simulink model "P1_Ex1"  (R2021a)
settings: Solver=FixedStepAuto  StartTime=0.0  StopTime=Total_time  RelTol=1e-3
PreLoadFcn:
  | PreLoad_P1_Ex1
StopFcn:
  | post_P1_Ex1
values from neighbouring files (symbols this model uses):
  Tg = 0.005    [PreLoad_P1_Ex1.m]
libraries: arduinolib x5, simulink x2
settings Model: SimulationMode=external  ExtModeTrigDuration=2  Creator=Eneko Lerma  LastModifiedBy=Control Automatic
settings SolverCC: AlgebraicLoopSolver=TrustRegion
settings DataIOCC: ReturnWorkspaceOutputs=off
settings OptimizationCC: EnhancedBackFolding=on  PassReuseOutputArgsAs=Individual arguments  MaxStackSize=64  OptimizeBlockOrder=speed  DifferentSizesBufferReuse=on  OptimizationCustomize=off  EfficientTunableParamExpr=on
settings DebuggingCC: ParameterPrecisionLossMsg=none  ParameterTunabilityLossMsg=error  SFMachineParentedDataDiag=warning  ArithmeticOperatorsInVariantConditions=warning
settings HardwareCC: ProdBitPerPointer=32  ProdBitPerSizeT=32  ProdBitPerPtrDiffT=32  ProdLargestAtomicInteger=Long  ProdLargestAtomicFloat=Double  ProdWordSize=32  ProdHWDeviceType=ARM Compatible->ARM Cortex
settings SFSimCC: SimUseLocalCustomCode=off  MATLABDynamicMemAlloc=off  CustomCodeUndefinedFunction=UseInterfaceOnly
settings RTWCC: SystemTargetFile=ert.tlc  HardwareBoard=Arduino Due  TemplateMakefile=ert_default_tmf  GenerateReport=on  RTWUseLocalCustomCode=off  Toolchain=Arduino ARM  BuildConfiguration=Faster Runs  IncludeHyperlinkInReport=on  LaunchReport=on  GenerateTraceInfo=on  GenerateTraceReport=on  GenerateTraceReportSl=on  GenerateTraceReportSf=on  GenerateTraceReportEml=on
settings RTWCC: CustomTerminator=|
  | writeDigitalPin((uint8_T)3, 0);
  | writeDigitalPin((uint8_T)5, 0);
settings CodeAppCC: ForceParamTrailComments=on  IgnoreCustomStorageClasses=off  OperatorAnnotations=on  SimulinkDataObjDesc=on  SFDataObjDesc=on  InsertBlockDesc=on
settings ERTTargetCC: SupportContinuousTime=on  SupportVariableSizeSignals=on

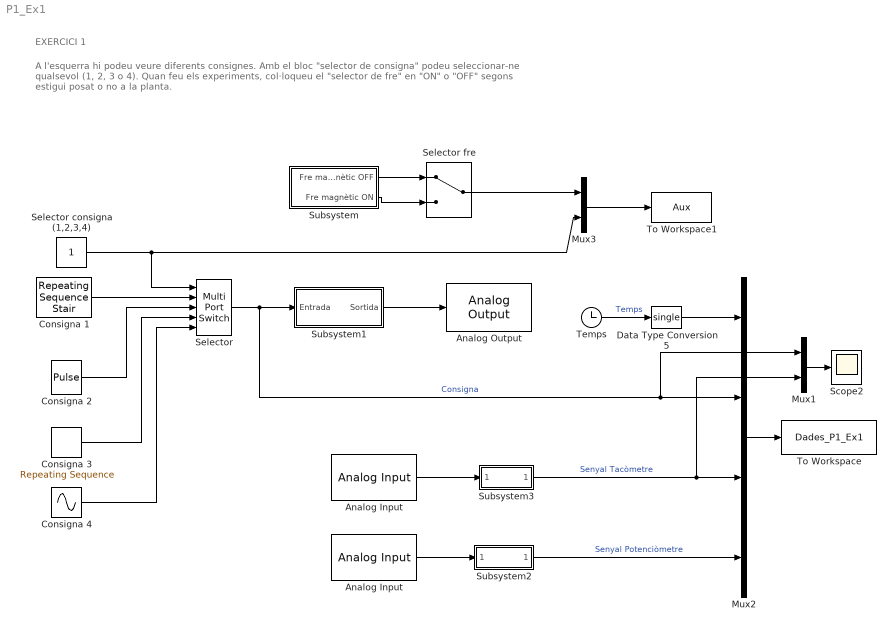
== system P1_Ex1 ==
  note: A l'esquerra hi podeu veure diferents consignes. Amb el bloc "selector de consigna" podeu seleccionar-ne
      | qualsevol (1, 2, 3 o 4). Quan feu els experiments, col·loqueu el "selector de fre" en "ON" o "OFF"
      | segons estigui posat o no a la planta.
  note: EXERCICI 1
  Analog Input : arduinolib/Analog Input  pinNumber=0  ReadResultsOnly=off  ConversionTriggerSource=Software  ExternalTriggerType=uint32(0)  OutputDataType=uint16  EnableConversionCompleteNotify=off  EnableOuputStatus=off  SampleTime=Tg  blockPlatform=arduino
  "Analog Input  " : arduinolib/Analog Input  pinNumber=1  ReadResultsOnly=off  ConversionTriggerSource=Software  ExternalTriggerType=uint32(0)  OutputDataType=uint16  EnableConversionCompleteNotify=off  EnableOuputStatus=off  SampleTime=Tg  blockPlatform=arduino
  Analog Output : arduinolib/Analog Output  DACpin=DAC1  blockPlatform=arduino
      settings: SourceProductBaseCode=ARDUINO
  Consigna 1 : simulink/Sources/Repeating Sequence Stair  OutValues=input_vector  tsamp=t  OutMin=[]  OutMax=[]  OutDataTypeStr=float('double')  OutputDataTypeScalingMode=Specify via dialog  OutDataType=float('double')  ConRadixGroup=Best Precision: Vector-wise  OutScaling=2^-12
  Consigna 2 : DiscretePulseGenerator  PulseType=Time based  Amplitude=5  Period=5  PulseWidth=50
  Consigna 3 : simulink/Sources/Repeating Sequence  rep_seq_t=[0 2.5]  rep_seq_y=[0 2]
  Consigna 4 : Sin  Amplitude=5  Frequency=2*pi*0.5  SampleTime=0
  Data Type Conversion5 : DataTypeConversion  OutDataTypeStr=single
  Mux1 : Mux  Inputs=2
  Mux2 : Mux
  Mux3 : Mux  Inputs=2
  Scope2 : Scope
  Selector : MultiPortSwitch  Inputs=4  OutDataTypeStr=single
  Selector consigna (1,2,3,4) : Constant
  Selector fre : ManualSwitch
  Subsystem : Subsystem
  Subsystem1 : Subsystem
  Subsystem2 : Subsystem
  Subsystem3 : Subsystem
  Temps : Clock
  To Workspace : ToWorkspace  VariableName=Dades_P1_Ex1  SampleTime=-1
  To Workspace1 : ToWorkspace  VariableName=Aux  SampleTime=-1
  wires:
  Selector consigna (1,2,3,4)/1 -> Mux3/2, Selector/1
  Consigna 3/1 -> Selector/4
  Consigna 4/1 -> Selector/5
  Consigna 2/1 -> Selector/3
  Consigna 1/1 -> Selector/2
  Mux3/1 -> To Workspace1/1
  Selector fre/1 -> Mux3/1
  Subsystem/1(Fre magnètic OFF) -> Selector fre/1
  Subsystem/2(Fre magnètic ON) -> Selector fre/2
  Data Type Conversion5/1 -> Mux2/1
  Temps/1 -> Data Type Conversion5/1  "Temps"
  Mux2/1 -> To Workspace/1
  Selector/1 -> Mux1/1, Mux2/2, Subsystem1/1(Entrada)  "Consigna"
  Subsystem1/1(Sortida) -> Analog Output/1
  "Analog Input  "/1 -> Subsystem2/1(" ")
  Subsystem2/1("    ") -> Mux2/4  "Senyal Potenciòmetre"
  Analog Input/1 -> Subsystem3/1("  ")
  Subsystem3/1("   ") -> Mux1/2, Mux2/3  "Senyal Tacòmetre"
  Mux1/1 -> Scope2/1

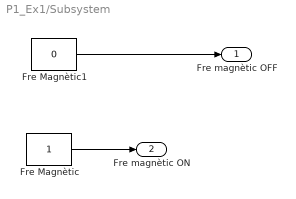
== system P1_Ex1/Subsystem ==
  Fre Magnètic : Constant  OutDataTypeStr=double
  Fre Magnètic1 : Constant  Value=0  OutDataTypeStr=double
  Fre magnètic OFF : Outport  VectorParamsAs1DForOutWhenUnconnected=off
  Fre magnètic ON : Outport  Port=2  VectorParamsAs1DForOutWhenUnconnected=off
  wires:
  Fre Magnètic1/1 -> Fre magnètic OFF/1
  Fre Magnètic/1 -> Fre magnètic ON/1

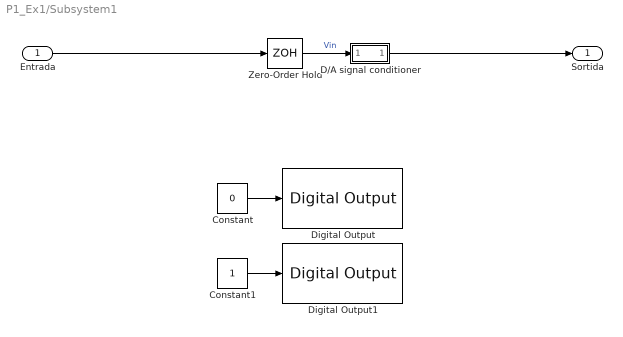
== system P1_Ex1/Subsystem1 ==
  Entrada : Inport
  Constant : Constant  Value=0
  Constant1 : Constant
  D/A signal conditioner : Subsystem
  Digital Output : arduinolib/Digital Output  pinNumber=3  Direction=output  blockPlatform=arduino
  Digital Output1 : arduinolib/Digital Output  pinNumber=5  Direction=output  blockPlatform=arduino
  Zero-Order Hold : ZeroOrderHold  SampleTime=Tg
  Sortida : Outport  VectorParamsAs1DForOutWhenUnconnected=off
  wires:
  Zero-Order Hold/1 -> D/A signal conditioner/1("  ")  "Vin"
  D/A signal conditioner/1(" ") -> Sortida/1
  Entrada/1 -> Zero-Order Hold/1
  Constant/1 -> Digital Output/1
  Constant1/1 -> Digital Output1/1

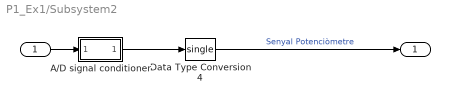
== system P1_Ex1/Subsystem2 ==
  " " : Inport
  "A/D signal conditioner  " : Subsystem
  Data Type Conversion4 : DataTypeConversion  OutDataTypeStr=single
  "    " : Outport  VectorParamsAs1DForOutWhenUnconnected=off
  wires:
  "A/D signal conditioner  "/1(" ") -> Data Type Conversion4/1
  Data Type Conversion4/1 -> "    "/1  "Senyal Potenciòmetre"
  " "/1 -> "A/D signal conditioner  "/1(" ")

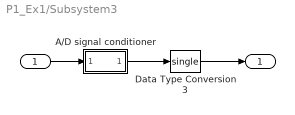
== system P1_Ex1/Subsystem3 ==
  "  " : Inport
  A/D signal conditioner : Subsystem
  Data Type Conversion3 : DataTypeConversion  OutDataTypeStr=single
  "   " : Outport  VectorParamsAs1DForOutWhenUnconnected=off
  wires:
  A/D signal conditioner/1(" ") -> Data Type Conversion3/1
  Data Type Conversion3/1 -> "   "/1
  "  "/1 -> A/D signal conditioner/1(" ")

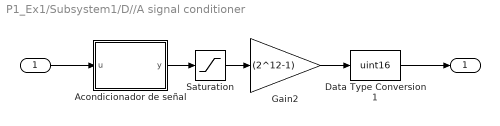
== system P1_Ex1/Subsystem1/D//A signal conditioner ==
  "  " : Inport  OutDataTypeStr=single
  Acondicionador de señal : MATLAB Function  TreatAsAtomicUnit=on
  Data Type Conversion1 : DataTypeConversion  OutDataTypeStr=uint16
  Gain2 : Gain  Gain=(2^12-1)  OutDataTypeStr=single
  Saturation : Saturate  UpperLimit=1  LowerLimit=0  OutDataTypeStr=single
  " " : Outport  OutDataTypeStr=uint16  VectorParamsAs1DForOutWhenUnconnected=off
  wires:
  Saturation/1 -> Gain2/1
  Data Type Conversion1/1 -> " "/1
  Acondicionador de señal/1(y) -> Saturation/1
  "  "/1 -> Acondicionador de señal/1(u)
  Gain2/1 -> Data Type Conversion1/1

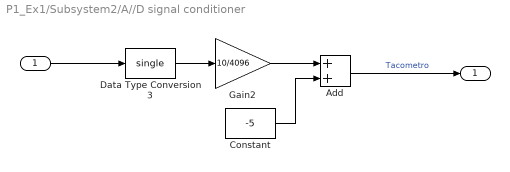
== system P1_Ex1/Subsystem2/A//D signal conditioner   ==
  " " : Inport
  Add : Sum  AccumDataTypeStr=single
  Constant : Constant  Value=-5  OutDataTypeStr=single
  Data Type Conversion3 : DataTypeConversion  OutDataTypeStr=single
  Gain2 : Gain  Gain=10/4096  OutDataTypeStr=single
  " " : Outport  VectorParamsAs1DForOutWhenUnconnected=off
  wires:
  Data Type Conversion3/1 -> Gain2/1
  Constant/1 -> Add/2
  Gain2/1 -> Add/1
  Add/1 -> " "/1  "Tacometro"
  " "/1 -> Data Type Conversion3/1

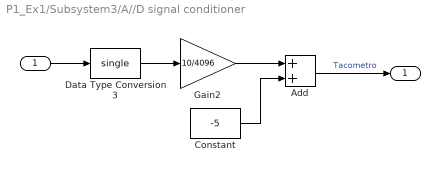
== system P1_Ex1/Subsystem3/A//D signal conditioner ==
  " " : Inport
  Add : Sum  AccumDataTypeStr=single
  Constant : Constant  Value=-5  OutDataTypeStr=single
  Data Type Conversion3 : DataTypeConversion  OutDataTypeStr=single
  Gain2 : Gain  Gain=10/4096  OutDataTypeStr=single
  " " : Outport  VectorParamsAs1DForOutWhenUnconnected=off
  wires:
  " "/1 -> Data Type Conversion3/1
  Add/1 -> " "/1  "Tacometro"
  Gain2/1 -> Add/1
  Constant/1 -> Add/2
  Data Type Conversion3/1 -> Gain2/1

== matlab function P1_Ex1/Subsystem1/D//A signal conditioner/Acondicionador de señal ==
  data: u input; y output
function y = fcn(u)
y =0.0968*u+0.5058;
